simulink model "soc_fpga"  (R2023b)
settings: Solver=FixedStepDiscrete  StartTime=0.0  StopTime=2e-06  RelTol=1e-3
libraries: hwlogicconnlib x2
settings Model: Creator=user poco smart  LastModifiedBy=user poco smart
settings SolverCC: AlgebraicLoopSolver=TrustRegion  PositivePriorityOrder=on  MinimalZcImpactIntegration=on
settings DataIOCC: SaveOutput=off  SaveTime=off  ReturnWorkspaceOutputs=off
settings OptimizationCC: DefaultParameterBehavior=Inlined  EnhancedBackFolding=on  PassReuseOutputArgsAs=Individual arguments  MaxStackSize=64  OptimizeBlockOrder=speed  DifferentSizesBufferReuse=on  OptimizationCustomize=off  EfficientTunableParamExpr=on
settings DebuggingCC: ParameterPrecisionLossMsg=none  ParameterTunabilityLossMsg=error  UnconnectedInputMsg=warning  UnconnectedOutputMsg=warning  UnconnectedLineMsg=warning  PregeneratedLibrarySubsystemCodeDiagnostic=none  ArithmeticOperatorsInVariantConditions=warning
settings HardwareCC: ProdBitPerPointer=32  ProdBitPerSizeT=32  ProdBitPerPtrDiffT=32  ProdLargestAtomicFloat=None  ProdIntDivRoundTo=Undefined  ProdEndianess=Unspecified  ProdWordSize=32  ProdHWDeviceType=ASIC/FPGA->ASIC/FPGA  TargetBitPerPointer=64  TargetBitPerSizeT=64  TargetBitPerPtrDiffT=64  TargetLongLongMode=on  TargetIntDivRoundTo=Zero  TargetEndianess=LittleEndian  TargetWordSize=64  TargetHWDeviceType=Custom Processor->MATLAB Host Computer  ProdEqTarget=off  HardwareBoardFeatureSet=SoCBlockset
settings ModelReferenceCC: EnableRefExpFcnMdlSchedulingChecks=on  ModelReferenceNumInstancesAllowed=Single
settings SFSimCC: SimUseLocalCustomCode=off  CustomCodeUndefinedFunction=UseInterfaceOnly
settings RTWCC: Description=Embedded Coder  SystemTargetFile=ert.tlc  HardwareBoard=ZedBoard  TLCOptions="-aInlineSetEventsForThisBaseRateFcn=TLC_FALSE -aSuppressMultiTaskScheduler=TLC_FALSE  -aRateBasedStepFcn=0"  TemplateMakefile=ert_default_tmf  GenerateReport=on  RTWUseLocalCustomCode=off  Toolchain=Linaro AArch32 Linux v6.3.1  IncludeHyperlinkInReport=on  LaunchReport=on  GenerateTraceInfo=on  GenerateTraceReport=on  GenerateTraceReportSl=on  GenerateTraceReportSf=on  GenerateTraceReportEml=on  DLArmComputeVersion=19.05
settings CodeAppCC: ForceParamTrailComments=on  IgnoreCustomStorageClasses=off  OperatorAnnotations=on  SimulinkDataObjDesc=on  SFDataObjDesc=on  InsertBlockDesc=on
settings ERTTargetCC: ExtModeTransport=2  ExtModeStaticAlloc=on  ExtModeMexFile=ext_xcp  ExtModeIntrfLevel=Level2 - Open
settings ConfigComp: CovBoundaryAbsTol=1.0e-5
settings SettingsController: UseSoCProfilerForTargets=0

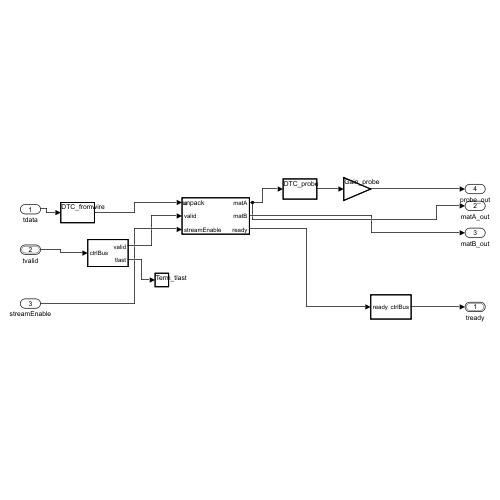
[thumbnail: Simulink's stored preview of the top-level diagram]
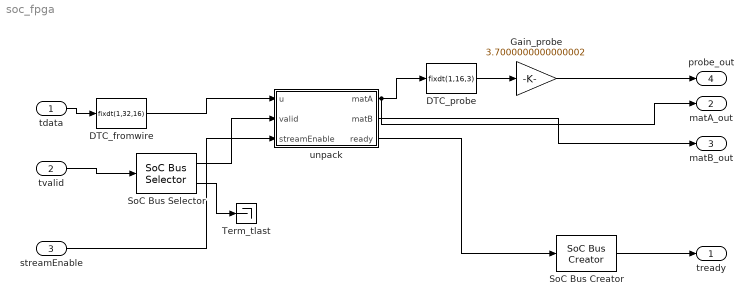
== system soc_fpga ==
  tdata : Inport  OutDataTypeStr=int32  PortDimensions=25
  tvalid : Inport  Port=2  OutDataTypeStr=Bus: StreamM2SBusObj  PortDimensions=1
  streamEnable : Inport  Port=3  OutDataTypeStr=boolean  PortDimensions=1
  DTC_fromwire : DataTypeConversion  OutDataTypeStr=fixdt(1,32,16)  ConvertRealWorld=Stored Integer (SI)  SaturateOnIntegerOverflow=off  RndMeth=Floor
  DTC_probe : DataTypeConversion  OutDataTypeStr=fixdt(1,16,3)  RndMeth=Floor
  Gain_probe : Gain  Gain=3.7000000000000002  OutDataTypeStr=fixdt(1,16,3)  SaturateOnIntegerOverflow=on
  SoC Bus Creator : hwlogicconnlib/SoC Bus Creator  Protocol=Data stream  ctrltype=Ready
  SoC Bus Selector : hwlogicconnlib/SoC Bus Selector  Protocol=Data stream  ctrltype=Valid
  Term_tlast : Terminator
  unpack : MATLAB Function  TreatAsAtomicUnit=on
  tready : Outport  OutDataTypeStr=Bus: StreamS2MBusObj
  matA_out : Outport  Port=2
  matB_out : Outport  Port=3
  probe_out : Outport  Port=4
  wires:
  tvalid/1 -> SoC Bus Selector/1
  SoC Bus Selector/1 -> unpack/2(valid)
  SoC Bus Selector/2 -> Term_tlast/1
  tdata/1 -> DTC_fromwire/1
  DTC_fromwire/1 -> unpack/1(u)
  streamEnable/1 -> unpack/3(streamEnable)
  unpack/1(matA) -> DTC_probe/1, matA_out/1
  DTC_probe/1 -> Gain_probe/1
  Gain_probe/1 -> probe_out/1
  unpack/2(matB) -> matB_out/1
  unpack/3(ready) -> SoC Bus Creator/1
  SoC Bus Creator/1 -> tready/1

== matlab function soc_fpga/unpack ==
  data: u input; matA output; valid input; streamEnable input; matB output; ready output
function [matA, matB, ready] = unpack(u, valid, streamEnable)
%#codegen
% GENERATO DA build_soc_fpga.m â€” non modificare a mano.
% Indici e forme provengono da soc_params (regola R2).
% Srotolamento column-major, coerente con ref_model.m.

    matA = reshape(u(1:9), [3 3]);
    matB = reshape(u(10:25), [4 4]);

    % Handshake.
    % ready NON deve dipendere da valid: e' la regola AXI4-Stream
    % (VALID non aspetta READY, READY non e' funzione di VALID).
    % Violarla produce uno stallo: il canale non alza valid finche'
    % non vede ready, e ready non sale perche' aspetta valid.
    % Misurato: tvalid.valid e tready.ready costantemente 0, uscite
    % della PL sempre nulle.
    % Resta un SEGNAPOSTO: sempre pronto = nessuna contropressione.
    ready = streamEnable;
    %#ok<INUSD> valid non usato di proposito
end
